simulink library "stonesoup_lib"  (R2025b)
settings: Solver=VariableStepAuto  StartTime=0.0  StopTime=10.0  RelTol=1e-3
settings Model: Creator=e  LastModifiedBy=e

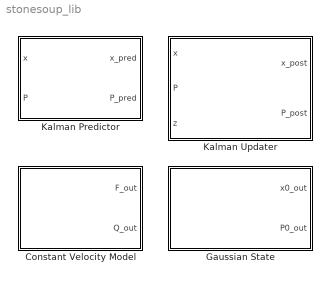
== system stonesoup_lib ==
  Constant Velocity Model : Subsystem  mask(Constant Velocity Model){ndim=2, dt=0.1, q=0.01}
      mask prompts: ndim "Spatial dimensions:"; dt "Time step (s):"; q "Process noise:"
      mask help: Generates F and Q for constant velocity motion
      mask init:
      | state_dim = 2 * ndim;
      | F_cv = eye(state_dim);
      | for i = 1:ndim, F_cv(2*i-1, 2*i) = dt; end
      | Q_block = [dt^3/3, dt^2/2; dt^2/2, dt] * q;
      | Q_cv = kron(eye(ndim), Q_block);
      mask Display:
      | color('red');
      | patch([0.1 0.9 0.9 0.1], [0.1 0.1 0.9 0.9], [1 0.9 0.9]);
      | text(0.5, 0.65, 'Constant', 'HorizontalAlignment', 'center', 'FontWeight', 'bold');
      | text(0.5, 0.35, 'Velocity', 'HorizontalAlignment', 'center');
      | port_label('output', 1, 'F');
      | port_label('output', 2, 'Q');
  Gaussian State : Subsystem  mask(Gaussian State Source){x0=[0; 0; 0; 0], P0=eye(4)}
      mask prompts: x0 "Initial state x0:"; P0 "Initial covariance P0:"
      mask help: Initial state and covariance for Kalman filter
      mask init:
      | x0_init = x0;
      | P0_init = P0;
      mask Display:
      | color('magenta');
      | patch([0.1 0.9 0.9 0.1], [0.1 0.1 0.9 0.9], [1 0.9 1]);
      | text(0.5, 0.65, 'Gaussian', 'HorizontalAlignment', 'center', 'FontWeight', 'bold');
      | text(0.5, 0.35, 'State', 'HorizontalAlignment', 'center');
      | port_label('output', 1, 'x_0');
      | port_label('output', 2, 'P_0');
  Kalman Predictor : Subsystem  mask(Kalman Predictor){F=eye(4), Q=0.01*eye(4)}
      mask prompts: F "Transition matrix F:"; Q "Process noise Q:"
      mask help: Kalman filter prediction: x_pred = F*x, P_pred = F*P*F' + Q
      mask Display:
      | color('blue');
      | patch([0.1 0.9 0.9 0.1], [0.1 0.1 0.9 0.9], [0.9 0.9 1]);
      | text(0.5, 0.65, 'Kalman', 'HorizontalAlignment', 'center', 'FontWeight', 'bold');
      | text(0.5, 0.35, 'Predictor', 'HorizontalAlignment', 'center');
      | port_label('input', 1, 'x');
      | port_label('input', 2, 'P');
      | port_label('output', 1, 'x_{pred}');
      | port_label('output', 2, 'P_{pred}');
  Kalman Updater : Subsystem  mask(Kalman Updater){H=[1 0 0 0; 0 0 1 0], R=0.1*eye(2)}
      mask prompts: H "Measurement matrix H:"; R "Measurement noise R:"
      mask help: Kalman filter update step with measurement
      mask Display:
      | color('green');
      | patch([0.1 0.9 0.9 0.1], [0.1 0.1 0.9 0.9], [0.9 1 0.9]);
      | text(0.5, 0.65, 'Kalman', 'HorizontalAlignment', 'center', 'FontWeight', 'bold');
      | text(0.5, 0.35, 'Updater', 'HorizontalAlignment', 'center');
      | port_label('input', 1, 'x');
      | port_label('input', 2, 'P');
      | port_label('input', 3, 'z');
      | port_label('output', 1, 'x_{post}');
      | port_label('output', 2, 'P_{post}');

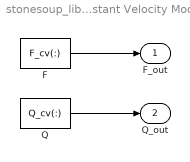
== system stonesoup_lib/Constant Velocity Model ==
  F : Constant  Value=F_cv(:)
  Q : Constant  Value=Q_cv(:)
  F_out : Outport
  Q_out : Outport  Port=2
  wires:
  F/1 -> F_out/1
  Q/1 -> Q_out/1

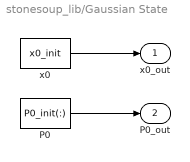
== system stonesoup_lib/Gaussian State ==
  P0 : Constant  Value=P0_init(:)
  x0 : Constant  Value=x0_init
  x0_out : Outport
  P0_out : Outport  Port=2
  wires:
  x0/1 -> x0_out/1
  P0/1 -> P0_out/1

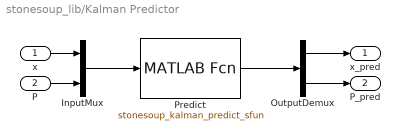
== system stonesoup_lib/Kalman Predictor ==
  x : Inport
  P : Inport  Port=2
  InputMux : Mux  Inputs=2
  OutputDemux : Demux  Outputs=2
  Predict : MATLABFcn  MATLABFcn=stonesoup_kalman_predict_sfun
  x_pred : Outport
  P_pred : Outport  Port=2
  wires:
  x/1 -> InputMux/1
  P/1 -> InputMux/2
  InputMux/1 -> Predict/1
  Predict/1 -> OutputDemux/1
  OutputDemux/1 -> x_pred/1
  OutputDemux/2 -> P_pred/1

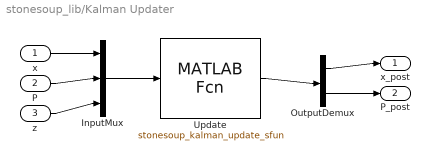
== system stonesoup_lib/Kalman Updater ==
  x : Inport
  P : Inport  Port=2
  z : Inport  Port=3
  InputMux : Mux  Inputs=3
  OutputDemux : Demux  Outputs=2
  Update : MATLABFcn  MATLABFcn=stonesoup_kalman_update_sfun
  x_post : Outport
  P_post : Outport  Port=2
  wires:
  x/1 -> InputMux/1
  P/1 -> InputMux/2
  z/1 -> InputMux/3
  InputMux/1 -> Update/1
  Update/1 -> OutputDemux/1
  OutputDemux/1 -> x_post/1
  OutputDemux/2 -> P_post/1
